simulink model "chap8_4sim"  (Simulink 5.1)
settings: Solver=ode45  SolverMode=SingleTasking  StartTime=0.0  StopTime=3  FixedStep=0.001  RelTol=1e-3
settings Model: LastModifiedBy=Administrator  ExtModeTrigMode=oneshot  ExtModeArmWhenConnect=off  LimitDataPoints=off  ProdHWDeviceType=Microprocessor

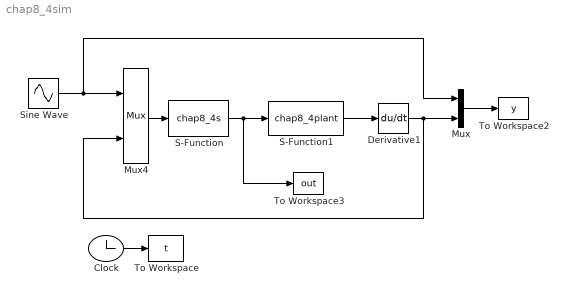
== system chap8_4sim ==
  Clock : Clock
  Derivative1 : Derivative
  Mux : Mux  Inputs=2
  Mux4 : Mux  Inputs=2
  S-Function : S-Function  FunctionName=chap8_4s
  S-Function1 : S-Function  FunctionName=chap8_4plant
  Sine Wave : Sin  Amplitude=0.5  Frequency=2*pi  SampleTime=0
  To Workspace : ToWorkspace  VariableName=t  SampleTime=-1  SaveFormat=Array
  To Workspace2 : ToWorkspace  VariableName=y  SampleTime=-1  SaveFormat=Array
  To Workspace3 : ToWorkspace  VariableName=out  SampleTime=-1  SaveFormat=Array
  wires:
  Mux4/1 -> S-Function/1
  Sine Wave/1 -> Mux/1, Mux4/1
  Mux/1 -> To Workspace2/1
  S-Function1/1 -> Derivative1/1
  Derivative1/1 -> Mux4/2, Mux/2
  Clock/1 -> To Workspace/1
  S-Function/1 -> S-Function1/1, To Workspace3/1
